simulink model "MIL4L3_SW6_V1_20220211"  (R2018b)
settings: Solver=FixedStepAuto  StartTime=0.0  StopTime=inf  FixedStep=0.001  RelTol=1e-3
PreLoadFcn:
  | A0_MILtest;
undefined symbols (not defined in the file or in its folder): Clb_ICADirect_LaneDisp_StateFive, Clb_ICADirect_LaneDisp_StateFour, Clb_ICADirect_LaneDisp_StateOne, Clb_ICADirect_LaneDisp_StateThree, Clb_ICADirect_LaneDisp_StateTwo, Clb_ICADirect_LaneDisp_StateZero, Clb_ICADirect_LaneDispSW, Clb_ICADirect_TrnLghtsCom_Switch, Clb_ICADirect_TrnLghtsCom_Value, Clb_ICADirect_TrnLghtsCrtl_Inhb, IMAP_Clb_ACU_Driver_Belt, IMAP_Clb_ACU_Driver_Belt_Over, IMAP_Clb_ACU_Passenger_Belt, IMAP_Clb_ACU_Passenger_Belt_Over, IMAP_Clb_ACU_RearLeft_Belt, IMAP_Clb_ACU_RearLeft_Belt_Over, IMAP_Clb_ACU_RearMiddle_Belt, IMAP_Clb_ACU_RearMiddle_Belt_Over, IMAP_Clb_ACU_RearRight_Belt, IMAP_Clb_ACU_RearRight_Belt_Over, IMAP_Clb_AEB_Switch, IMAP_Clb_AEB_Switch_Over, IMAP_Clb_ALC_TLC_Mode, IMAP_Clb_ALC_TLC_Mode_Over, IMAP_Clb_BCM_Battery_Voltage, IMAP_Clb_BCM_Battery_Voltage_Over, IMAP_Clb_BCM_BrakeLamp_State, IMAP_Clb_BCM_BrakeLamp_State_Over, IMAP_Clb_BCM_CHMSL_Status, IMAP_Clb_BCM_CHMSL_Status_Over, IMAP_Clb_BCM_Door_Lock_State, IMAP_Clb_BCM_Door_Lock_State_Over, IMAP_Clb_BCM_FrontWiper_State, IMAP_Clb_BCM_FrontWiper_State_Over, IMAP_Clb_BCM_FrontWiper_Switch, IMAP_Clb_BCM_FrontWiper_Switch_Over, IMAP_Clb_BCM_HazardLamp, IMAP_Clb_BCM_HazardLamp_Over, IMAP_Clb_BCM_HazardLamp_Switch, IMAP_Clb_BCM_HazardLamp_Switch_Over, IMAP_Clb_BCM_HighBeam_State, IMAP_Clb_BCM_HighBeam_State_Over, IMAP_Clb_BCM_Ignition_State, IMAP_Clb_BCM_Ignition_State_Over, IMAP_Clb_BCM_IHBC_Enabled, IMAP_Clb_BCM_IHBC_Enabled_Over, IMAP_Clb_BCM_Left_Light, IMAP_Clb_BCM_Left_Light_Over, IMAP_Clb_BCM_LeftTurn_Switch, IMAP_Clb_BCM_LeftTurn_Switch_Over, IMAP_Clb_BCM_LF_Door_State, IMAP_Clb_BCM_LF_Door_State_Over, IMAP_Clb_BCM_LowBeam_State, IMAP_Clb_BCM_LowBeam_State_Over, IMAP_Clb_BCM_LR_Door_State, IMAP_Clb_BCM_LR_Door_State_Over, IMAP_Clb_BCM_RF_Door_State, IMAP_Clb_BCM_RF_Door_State_Over, IMAP_Clb_BCM_Right_Light, IMAP_Clb_BCM_Right_Light_Over ... (+547)
libraries: CarMaker4SL x2153, simulink x292, dspstat3 x3, canmsglib x2, simulink_extras x1
(part 14 of 52)

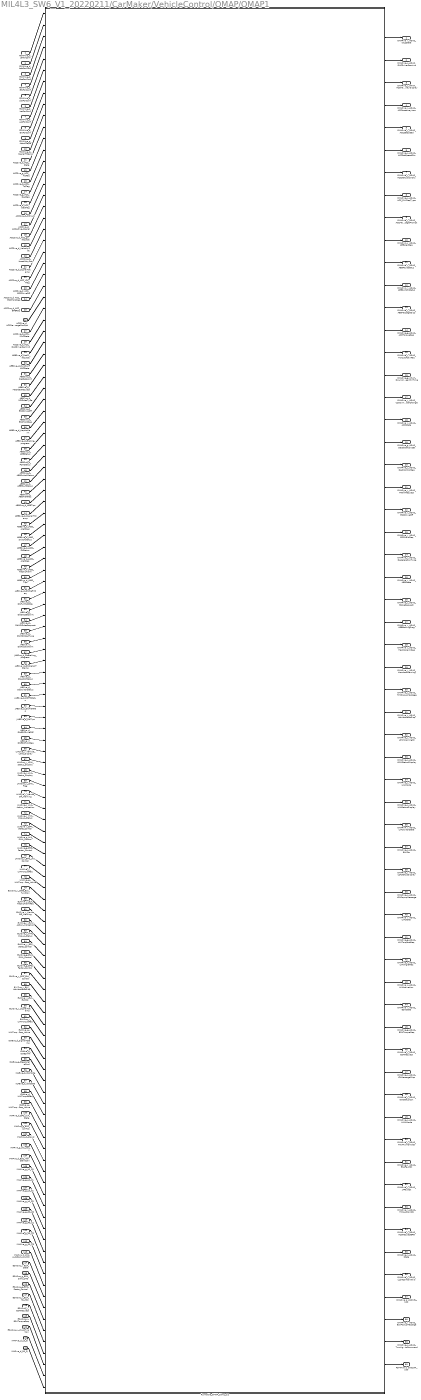
== system MIL4L3_SW6_V1_20220211/CarMaker/VehicleControl/OMAP/OMAP1 ==
  FDMMve_d_JaFcnConf : Inport  OutDataTypeStr=UInt16  PortDimensions=1
  FDMMve_d_AebFcnConf : Inport  Port=2  OutDataTypeStr=UInt16  PortDimensions=1
  FDMMve_d_EsaFcnConf : Inport  Port=3  OutDataTypeStr=UInt16  PortDimensions=1
  FDMMve_d_ElkFcnConf : Inport  Port=4  OutDataTypeStr=UInt16  PortDimensions=1
  FDMMve_d_LkaFcnConf : Inport  Port=5  OutDataTypeStr=UInt16  PortDimensions=1
  FDMMve_d_IcaFcnConf : Inport  Port=6  OutDataTypeStr=UInt16  PortDimensions=1
  FDMMve_d_AccFcnConf : Inport  Port=7  OutDataTypeStr=UInt16  PortDimensions=1
  FDMMve_d_EwFcnConf : Inport  Port=8  OutDataTypeStr=UInt16  PortDimensions=1
  FDMMve_g_Adas2Fapa : Inport  Port=9  OutDataTypeStr=UInt32  PortDimensions=1
  FDMMve_d_SignalTStamp : Inport  Port=10  OutDataTypeStr=UInt16  PortDimensions=1
  ACCSve_d_ACC_State : Inport  Port=11  OutDataTypeStr=UInt16  PortDimensions=1
  ACCSve_g_ACC_TqReq : Inport  Port=12  OutDataTypeStr=T_M_Nm_Float32  PortDimensions=1
  ACCSve_d_ACC_TqFlag : Inport  Port=13  OutDataTypeStr=UInt16  PortDimensions=1
  ACCSve_g_ACC_DecReq : Inport  Port=14  OutDataTypeStr=T_M_Nm_Float32  PortDimensions=1
  ACCSve_d_ACC_DecFlag : Inport  Port=15  OutDataTypeStr=UInt16  PortDimensions=1
  ACCSve_d_CIPV_ID : Inport  Port=16  OutDataTypeStr=UInt16  PortDimensions=1
  ACCSve_d_ACCActive_Signal : Inport  Port=17  OutDataTypeStr=UInt16  PortDimensions=1
  ACCSve_d_ACC_go_request : Inport  Port=18  OutDataTypeStr=UInt16  PortDimensions=1
  ACCSve_d_VelocitySet : Inport  Port=19  OutDataTypeStr=UInt16  PortDimensions=1
  ACCSve_d_HeadWaySet : Inport  Port=20  OutDataTypeStr=UInt16  PortDimensions=1
  ACCSve_d_SignalTStamp : Inport  Port=21  OutDataTypeStr=UInt16  PortDimensions=1
  ACCSve_d_ACC_ICA_Flag : Inport  Port=22  OutDataTypeStr=UInt16  PortDimensions=1
  ACCSve_d_ACC_ESCDriveOff : Inport  Port=23  OutDataTypeStr=UInt16  PortDimensions=1
  ACCSve_d_ACC_ESCHoldReq : Inport  Port=24  OutDataTypeStr=UInt16  PortDimensions=1
  ACCSve_d_ACC_EPBReq : Inport  Port=25  OutDataTypeStr=UInt16  PortDimensions=1
  ACCSve_d_ACCMessagePrompt : Inport  Port=26  OutDataTypeStr=UInt16
  ACCSve_d_ACC_ISLCState : Inport  Port=27  OutDataTypeStr=UInt16  PortDimensions=1
  ACCSve_d_ACC_ISLCDriverRemind : Inport  Port=28  OutDataTypeStr=UInt16  PortDimensions=1
  AEBSve_d_Prefill_request : Inport  Port=29  OutDataTypeStr=UInt16  PortDimensions=1
  AEBSve_d_functionFARCState : Inport  Port=30  OutDataTypeStr=UInt16  PortDimensions=1
  AEBSve_g_DecSetpoint : Inport  Port=31  OutDataTypeStr=T_M_Nm_Float32  PortDimensions=1
  AEBSve_d_MDDdecRequest : Inport  Port=32  OutDataTypeStr=UInt16  PortDimensions=1
  AEBSve_d_MDDdecType : Inport  Port=33  OutDataTypeStr=UInt16  PortDimensions=1
  AEBSve_d_ESCDriveOff : Inport  Port=34  OutDataTypeStr=UInt16  PortDimensions=1
  AEBSve_d_ESCHoldReq : Inport  Port=35  OutDataTypeStr=UInt16  PortDimensions=1
  AEBSve_d_HapticAlarm : Inport  Port=36  OutDataTypeStr=UInt16  PortDimensions=1
  AEBSve_d_Braking_progress : Inport  Port=37  OutDataTypeStr=UInt16  PortDimensions=1
  AEBSve_d_AEBStatus : Inport  Port=38  OutDataTypeStr=UInt16  PortDimensions=1
  AEBSve_d_FCWStatus : Inport  Port=39  OutDataTypeStr=UInt16  PortDimensions=1
  AEBSve_d_AEBSwitchStatus : Inport  Port=40  OutDataTypeStr=UInt16  PortDimensions=1
  AEBSve_d_AEBFaultStatus : Inport  Port=41  OutDataTypeStr=UInt16  PortDimensions=1
  AEBSve_d_AEBAlertReq : Inport  Port=42  OutDataTypeStr=UInt16  PortDimensions=1
  AEBSve_d_AEBTips : Inport  Port=43  OutDataTypeStr=UInt16  PortDimensions=1
  AEBSve_d_SignalTStamp : Inport  Port=44  OutDataTypeStr=UInt16  PortDimensions=1
  AEBSve_d_JABS_AlertSign : Inport  Port=45  OutDataTypeStr=UInt16  PortDimensions=1
  AEBSve_d_JABS_SwitchStatus : Inport  Port=46  OutDataTypeStr=UInt16  PortDimensions=1
  AEBSve_d_JABS_FltStatus : Inport  Port=47  OutDataTypeStr=UInt16  PortDimensions=1
  AEBSve_d_JABS_AlertReq : Inport  Port=48  OutDataTypeStr=UInt16  PortDimensions=1
  AEBSve_d_JABS_HapticAlarm : Inport  Port=49  OutDataTypeStr=UInt16  PortDimensions=1
  AEBSve_d_JABS_Tips : Inport  Port=50  OutDataTypeStr=UInt16  PortDimensions=1
  JABSve_d_DbPrefillReq : Inport  Port=51  OutDataTypeStr=UInt16  PortDimensions=1
  JABSve_d_DbFunFARCSta : Inport  Port=52  OutDataTypeStr=UInt16  PortDimensions=1
  JABSve_g_DbDecSetpoint : Inport  Port=53  OutDataTypeStr=T_M_Nm_Float32  PortDimensions=1
  JABSve_d_DbMDDdecRequest : Inport  Port=54  OutDataTypeStr=UInt16  PortDimensions=1
  JABSve_d_DbMDDdecType : Inport  Port=55  OutDataTypeStr=UInt16  PortDimensions=1
  JABSve_d_DbHapticAlarm : Inport  Port=56  OutDataTypeStr=UInt16  PortDimensions=1
  JABSve_d_DbBraking_progress : Inport  Port=57  OutDataTypeStr=UInt16  PortDimensions=1
  JABSve_d_DbSignalTStamp : Inport  Port=58  OutDataTypeStr=UInt16  PortDimensions=1
  JABSve_d_DbJACWStatus : Inport  Port=59  OutDataTypeStr=UInt16  PortDimensions=1
  JABSve_d_DbSwitchStatus : Inport  Port=60  OutDataTypeStr=UInt16  PortDimensions=1
  JABSve_d_DbFltStatus : Inport  Port=61  OutDataTypeStr=UInt16  PortDimensions=1
  JABSve_d_DbAlertReq : Inport  Port=62  OutDataTypeStr=UInt16  PortDimensions=1
  JABSve_d_DbTips : Inport  Port=63  OutDataTypeStr=UInt16  PortDimensions=1
  JABSve_d_DbESCDriveOff : Inport  Port=64  OutDataTypeStr=UInt16  PortDimensions=1
  JABSve_d_DbESCHoldReq : Inport  Port=65  OutDataTypeStr=UInt16  PortDimensions=1
  LKASve_y_Vehicle_Lane_Display : Inport  Port=66  OutDataTypeStr=UInt8  PortDimensions=1
  LKASve_y_LDW_Status_Display : Inport  Port=67  OutDataTypeStr=UInt8  PortDimensions=1
  LKASve_y_LKA_Status_Display : Inport  Port=68  OutDataTypeStr=UInt8  PortDimensions=1
  LKASve_y_LDW_Flag : Inport  Port=69  OutDataTypeStr=UInt8  PortDimensions=1
  LKASve_y_Hands_Off_Warning : Inport  Port=70  OutDataTypeStr=UInt8  PortDimensions=1
  LKASve_y_LKA_Action_Indication : Inport  Port=71  OutDataTypeStr=UInt8  PortDimensions=1
  LKASve_y_HMI_Popup_Status : Inport  Port=72  OutDataTypeStr=UInt8  PortDimensions=1
  LKASve_y_EPS_State_Control : Inport  Port=73  OutDataTypeStr=UInt8  PortDimensions=1
  LKASve_g_LKA_SWA_Control : Inport  Port=74  OutDataTypeStr=T_M_Nm_Float32  PortDimensions=1
  LKASve_g_EPS_Factor_Control : Inport  Port=75  OutDataTypeStr=T_M_Nm_Float32  PortDimensions=1
  LKASve_y_EPS_LKA_Control : Inport  Port=76  OutDataTypeStr=UInt8  PortDimensions=1
  LKASve_y_LKATorqueReq : Inport  Port=77  OutDataTypeStr=UInt8  PortDimensions=1
  LKASve_g_LKATorqueReq_Value : Inport  Port=78  OutDataTypeStr=T_M_Nm_Float32  PortDimensions=1
  ELKSve_y_state_ELK_function : Inport  Port=79  OutDataTypeStr=UInt8  PortDimensions=1
  ELKSve_y_ELK_HapticAlarmReq : Inport  Port=80  OutDataTypeStr=UInt8  PortDimensions=1
  ELKSve_y_Hands_Off_Warning : Inport  Port=81  OutDataTypeStr=UInt8  PortDimensions=1
  ELKSve_y_ELK_Action_Indication : Inport  Port=82  OutDataTypeStr=UInt8  PortDimensions=1
  ELKSve_y_HMI_Popup_Status : Inport  Port=83  OutDataTypeStr=UInt8  PortDimensions=1
  ELKSve_y_EPS_State_Control : Inport  Port=84  OutDataTypeStr=UInt8  PortDimensions=1
  ELKSve_g_ELK_SWA_Control : Inport  Port=85  OutDataTypeStr=T_M_Nm_Float32  PortDimensions=1
  ELKSve_g_EPS_Factor_Control : Inport  Port=86  OutDataTypeStr=T_M_Nm_Float32  PortDimensions=1
  ELKSve_y_EPS_ELK_Control : Inport  Port=87  OutDataTypeStr=UInt8  PortDimensions=1
  ELKSve_y_ELK_VehicleLaneDisp : Inport  Port=88  OutDataTypeStr=UInt8  PortDimensions=1
  ELKSve_y_ELK_ELKSts : Inport  Port=89  OutDataTypeStr=UInt8  PortDimensions=1
  ELKSve_y_SignalTStamp : Inport  Port=90  OutDataTypeStr=UInt8  PortDimensions=1
  ELKSve_y_LKATorqueReq : Inport  Port=91  OutDataTypeStr=UInt8  PortDimensions=1
  ELKSve_g_LKATorqueReq_Value : Inport  Port=92  OutDataTypeStr=T_M_Nm_Float32  PortDimensions=1
  ICABve_d_SignalTStamp : Inport  Port=93  OutDataTypeStr=UInt16  PortDimensions=1
  ICABva_d_ICAB2HMI : Inport  Port=94  OutDataTypeStr=UInt16  PortDimensions=20
  ICABve_g_SteerAngleCmd : Inport  Port=95  OutDataTypeStr=T_M_Nm_Float32  PortDimensions=1
  ICABve_d_ICAMode : Inport  Port=96  OutDataTypeStr=UInt16  PortDimensions=1
  ICABve_d_ICAState : Inport  Port=97  OutDataTypeStr=UInt16  PortDimensions=1
  ICABve_d_LKATorqueReq : Inport  Port=98  OutDataTypeStr=UInt16  PortDimensions=1
  ICABve_g_LKATorqueReq_Value : Inport  Port=99  OutDataTypeStr=T_M_Nm_Float32  PortDimensions=1
  IMAPve_d_EPS_LKA_State : Inport  Port=100  OutDataTypeStr=UInt16  PortDimensions=1
  IMAPve_g_ESC_LonAcc : Inport  Port=101  OutDataTypeStr=T_M_Nm_Float32  PortDimensions=1
  IMAPva_d_obj_id : Inport  Port=102  OutDataTypeStr=UInt16  PortDimensions=40
  IMAPva_g_obj_pos_x : Inport  Port=103  OutDataTypeStr=T_M_Nm_Float32  PortDimensions=40
  IMAPve_d_ESC_Veh_Standstill : Inport  Port=104  OutDataTypeStr=UInt16  PortDimensions=1
  IMAPve_g_L0_C0 : Inport  Port=105  OutDataTypeStr=T_M_Nm_Float32  PortDimensions=1
  IMAPve_g_L0_C1 : Inport  Port=106  OutDataTypeStr=T_M_Nm_Float32  PortDimensions=1
  IMAPve_g_L0_C2 : Inport  Port=107  OutDataTypeStr=T_M_Nm_Float32  PortDimensions=1
  IMAPve_g_L0_C3 : Inport  Port=108  OutDataTypeStr=T_M_Nm_Float32  PortDimensions=1
  IMAPve_g_R0_C0 : Inport  Port=109  OutDataTypeStr=T_M_Nm_Float32  PortDimensions=1
  IMAPve_g_R0_C1 : Inport  Port=110  OutDataTypeStr=T_M_Nm_Float32  PortDimensions=1
  IMAPve_g_R0_C2 : Inport  Port=111  OutDataTypeStr=T_M_Nm_Float32  PortDimensions=1
  IMAPve_g_R0_C3 : Inport  Port=112  OutDataTypeStr=T_M_Nm_Float32  PortDimensions=1
  IMAPve_d_APA_AutoPark_WorkSt : Inport  Port=113  OutDataTypeStr=UInt16  PortDimensions=1
  ESASve_y_ESA_State : Inport  Port=114  OutDataTypeStr=UInt8
  ESASve_g_ESA_SWA_CMD : Inport  Port=115  OutDataTypeStr=T_M_Nm_Float32
  ESASve_g_EPS_Factor_Control : Inport  Port=116  OutDataTypeStr=T_M_Nm_Float32
  ESASve_y_ESA_FaultSt : Inport  Port=117  OutDataTypeStr=UInt8
  ESASve_y_ESARequest : Inport  Port=118  OutDataTypeStr=UInt8
  ESASve_y_ESATorqueReq : Inport  Port=119  OutDataTypeStr=T_M_Nm_Float32
  ESASve_y_LKAActivation : Inport  Port=120  OutDataTypeStr=UInt8
  IMAPve_d_L0_Q : Inport  Port=121  OutDataTypeStr=UInt16
  IMAPve_d_R0_Q : Inport  Port=122  OutDataTypeStr=UInt16
  Runnable_OMAP_10ms_sys : Subsystem
  OMAPve_y_ADAS_ISLCState : Outport  OutDataTypeStr=UInt8  PortDimensions=1
  OMAPve_y_ADAS_ISLCDriverRemind : Outport  Port=2  OutDataTypeStr=UInt8  PortDimensions=1
  OMAPve_y_ADAS_ACCHeadwayDisplay : Outport  Port=3  OutDataTypeStr=UInt8  PortDimensions=1
  OMAPve_y_ADAS_ACCHeadwayIcon : Outport  Port=4  OutDataTypeStr=UInt8  PortDimensions=1
  OMAPve_y_ADAS_ACCSetSpeed : Outport  Port=5  OutDataTypeStr=UInt8  PortDimensions=1
  OMAPve_y_ADAS_ACCSetSpeedDis : Outport  Port=6  OutDataTypeStr=UInt8  PortDimensions=1
  OMAPve_y_ADAS_ACCStatusIconDis : Outport  Port=7  OutDataTypeStr=UInt8  PortDimensions=1
  OMAPve_y_ADAS_ACC_RVVReqType : Outport  Port=8  OutDataTypeStr=UInt8  PortDimensions=1
  OMAPve_y_ADAS_ACCMessagePrompt : Outport  Port=9  OutDataTypeStr=UInt8  PortDimensions=1
  OMAPve_y_ADAS_AEBAlertReq : Outport  Port=10  OutDataTypeStr=UInt8  PortDimensions=1
  OMAPve_y_ADAS_AEBFaultStatus : Outport  Port=11  OutDataTypeStr=UInt8  PortDimensions=1
  OMAPve_y_ADAS_AEBSwitchStatus : Outport  Port=12  OutDataTypeStr=UInt8  PortDimensions=1
  OMAPve_y_ADAS_AEBMassageDisp : Outport  Port=13  OutDataTypeStr=UInt8  PortDimensions=1
  OMAPve_g_ADAS_ACCTorqueReq : Outport  Port=14  OutDataTypeStr=T_M_Nm_Float32  PortDimensions=1
  OMAPve_y_ADAS_TorqueActivReq : Outport  Port=15  OutDataTypeStr=UInt8  PortDimensions=1
  OMAPve_g_ADAS_DownorUpGearMinTime : Outport  Port=16  OutDataTypeStr=T_M_Nm_Float32  PortDimensions=1
  OMAPve_y_ADAS_UpDownGearChange : Outport  Port=17  OutDataTypeStr=UInt8  PortDimensions=1
  OMAPve_y_ADAS_ACCState : Outport  Port=18  OutDataTypeStr=UInt8  PortDimensions=1
  OMAPve_g_ADAS_DecelerationSet : Outport  Port=19  OutDataTypeStr=T_M_Nm_Float32  PortDimensions=1
  OMAPve_y_ADAS_DeclControlReq : Outport  Port=20  OutDataTypeStr=UInt8  PortDimensions=1
  OMAPve_y_ADAS_PrefillRequest : Outport  Port=21  OutDataTypeStr=UInt8  PortDimensions=1
  OMAPve_y_ADAS_ESCDriveOff : Outport  Port=22  OutDataTypeStr=UInt8  PortDimensions=1
  OMAPve_y_ADAS_ESCHoldReq : Outport  Port=23  OutDataTypeStr=UInt8  PortDimensions=1
  OMAPve_y_ADAS_DecelerationType : Outport  Port=24  OutDataTypeStr=UInt8  PortDimensions=1
  OMAPve_y_ADAS_AEBState : Outport  Port=25  OutDataTypeStr=UInt8  PortDimensions=1
  OMAPve_y_ADAS_BrakeRequest : Outport  Port=26  OutDataTypeStr=UInt8  PortDimensions=1
  OMAPve_y_ADAS_AEBBrakingProg : Outport  Port=27  OutDataTypeStr=UInt8  PortDimensions=1
  OMAPve_y_ADAS_HapticAlarmReq : Outport  Port=28  OutDataTypeStr=UInt8  PortDimensions=1
  OMAPve_y_ADAS_Handsoffwarning : Outport  Port=29  OutDataTypeStr=UInt8  PortDimensions=1
  OMAPve_y_ADAS_HMIPopupMassage : Outport  Port=30  OutDataTypeStr=UInt8  PortDimensions=1
  OMAPve_y_ADAS_VehicleLaneDisp : Outport  Port=31  OutDataTypeStr=UInt8  PortDimensions=1
  OMAPve_y_ADAS_LDWWarningSt : Outport  Port=32  OutDataTypeStr=UInt8  PortDimensions=1
  OMAPve_y_ADAS_LDWStatusDisplay : Outport  Port=33  OutDataTypeStr=UInt8  PortDimensions=1
  OMAPve_y_ADAS_LKAMode : Outport  Port=34  OutDataTypeStr=UInt8  PortDimensions=1
  OMAPve_y_ADAS_LKAStatusDisplay : Outport  Port=35  OutDataTypeStr=UInt8  PortDimensions=1
  OMAPve_y_ADAS_LKASwitchState : Outport  Port=36  OutDataTypeStr=UInt8  PortDimensions=1
  OMAPve_y_ADAS_ELKSts : Outport  Port=37  OutDataTypeStr=UInt8  PortDimensions=1
  OMAPve_y_ADAS_LCAStatusDisplay : Outport  Port=38  OutDataTypeStr=UInt8  PortDimensions=1
  OMAPve_y_ADAS_LCAPopupMessage : Outport  Port=39  OutDataTypeStr=UInt8  PortDimensions=1
  OMAPve_y_ADAS_LKAState : Outport  Port=40  OutDataTypeStr=UInt8  PortDimensions=1
  OMAPve_g_ADAS_LKATorqFactReq : Outport  Port=41  OutDataTypeStr=T_M_Nm_Float32  PortDimensions=1
  OMAPve_g_ADAS_LKAAngleReq : Outport  Port=42  OutDataTypeStr=T_M_Nm_Float32  PortDimensions=1
  OMAPve_y_ADAS_LKAActivation : Outport  Port=43  OutDataTypeStr=UInt8  PortDimensions=1
  OMAPve_y_ADAS_ESAState : Outport  Port=44  OutDataTypeStr=UInt8  PortDimensions=1
  OMAPve_g_ADAS_ESATorqueReq : Outport  Port=45  OutDataTypeStr=T_M_Nm_Float32  PortDimensions=1
  OMAPve_y_ADAS_ESARequest : Outport  Port=46  OutDataTypeStr=UInt8  PortDimensions=1
  OMAPve_y_ADAS_ICAMassageDisp : Outport  Port=47  OutDataTypeStr=UInt8  PortDimensions=1
  OMAPve_y_ADAS_ICAStatusIcon : Outport  Port=48  OutDataTypeStr=UInt8  PortDimensions=1
  OMAPve_y_ADAS_HWAMode : Outport  Port=49  OutDataTypeStr=UInt8  PortDimensions=1
  OMAPve_y_ADAS_HWATurnOnIdctr : Outport  Port=50  OutDataTypeStr=UInt8  PortDimensions=1
  OMAPve_y_ADAS_ESAFaultSt : Outport  Port=51  OutDataTypeStr=UInt8  PortDimensions=1
  OMAPve_y_ADAS_JAFaultSt : Outport  Port=52  OutDataTypeStr=UInt8  PortDimensions=1
  OMAPve_y_ADAS_HWAActionSts : Outport  Port=53  OutDataTypeStr=UInt8  PortDimensions=1
  OMAPve_y_ADAS_ACCRequestEPB : Outport  Port=54  OutDataTypeStr=UInt8  PortDimensions=1
  OMAPve_y_ADAS_State : Outport  Port=55  OutDataTypeStr=UInt8  PortDimensions=1
  OMAPve_y_ADAS_LightControlValid : Outport  Port=56  OutDataTypeStr=UInt8  PortDimensions=1
  OMAPve_g_ob019L_100 : Outport  Port=57  OutDataTypeStr=UInt32  PortDimensions=1
  OMAPve_y_ADAS_ELKPopupMessage : Outport  Port=58  OutDataTypeStr=UInt8
  OMAPve_y_ADAS_TurnLightsCommand : Outport  Port=59  OutDataTypeStr=UInt8
  FDMMve_g_ob019H_100 : Outport  Port=60  OutDataTypeStr=UInt32
  wires:
  JABSve_d_DbTips/1 -> Runnable_OMAP_10ms_sys/63(JABSve_d_DbTips)
  ELKSve_y_ELK_VehicleLaneDisp/1 -> Runnable_OMAP_10ms_sys/88(ELKSve_y_ELK_VehicleLaneDisp)
  Runnable_OMAP_10ms_sys/39(OMAPve_y_ADAS_LCAPopupMessage) -> OMAPve_y_ADAS_LCAPopupMessage/1
  LKASve_g_LKATorqueReq_Value/1 -> Runnable_OMAP_10ms_sys/78(LKASve_g_LKATorqueReq_Value)
  ACCSve_d_SignalTStamp/1 -> Runnable_OMAP_10ms_sys/21(ACCSve_d_SignalTStamp)
  Runnable_OMAP_10ms_sys/18(OMAPve_y_ADAS_ACCState) -> OMAPve_y_ADAS_ACCState/1
  Runnable_OMAP_10ms_sys/24(OMAPve_y_ADAS_DecelerationType) -> OMAPve_y_ADAS_DecelerationType/1
  ACCSve_d_ACC_ISLCDriverRemind/1 -> Runnable_OMAP_10ms_sys/28(ACCSve_d_ACC_ISLCDriverRemind)
  AEBSve_d_MDDdecType/1 -> Runnable_OMAP_10ms_sys/33(AEBSve_d_MDDdecType)
  LKASve_y_LKA_Status_Display/1 -> Runnable_OMAP_10ms_sys/68(LKASve_y_LKA_Status_Display)
  Runnable_OMAP_10ms_sys/17(OMAPve_y_ADAS_UpDownGearChange) -> OMAPve_y_ADAS_UpDownGearChange/1
  Runnable_OMAP_10ms_sys/60(FDMMve_g_ob019H_100) -> FDMMve_g_ob019H_100/1
  Runnable_OMAP_10ms_sys/6(OMAPve_y_ADAS_ACCSetSpeedDis) -> OMAPve_y_ADAS_ACCSetSpeedDis/1
  IMAPve_d_L0_Q/1 -> Runnable_OMAP_10ms_sys/121(IMAPve_d_L0_Q)
  Runnable_OMAP_10ms_sys/58(OMAPve_y_ADAS_ELKPopupMessage) -> OMAPve_y_ADAS_ELKPopupMessage/1
  Runnable_OMAP_10ms_sys/11(OMAPve_y_ADAS_AEBFaultStatus) -> OMAPve_y_ADAS_AEBFaultStatus/1
  ESASve_g_ESA_SWA_CMD/1 -> Runnable_OMAP_10ms_sys/115(ESASve_g_ESA_SWA_CMD)
  Runnable_OMAP_10ms_sys/41(OMAPve_g_ADAS_LKATorqFactReq) -> OMAPve_g_ADAS_LKATorqFactReq/1
  Runnable_OMAP_10ms_sys/45(OMAPve_g_ADAS_ESATorqueReq) -> OMAPve_g_ADAS_ESATorqueReq/1
  ICABve_g_LKATorqueReq_Value/1 -> Runnable_OMAP_10ms_sys/99(ICABve_g_LKATorqueReq_Value)
  Runnable_OMAP_10ms_sys/46(OMAPve_y_ADAS_ESARequest) -> OMAPve_y_ADAS_ESARequest/1
  ESASve_y_ESARequest/1 -> Runnable_OMAP_10ms_sys/118(ESASve_y_ESARequest)
  ELKSve_y_Hands_Off_Warning/1 -> Runnable_OMAP_10ms_sys/81(ELKSve_y_Hands_Off_Warning)
  Runnable_OMAP_10ms_sys/20(OMAPve_y_ADAS_DeclControlReq) -> OMAPve_y_ADAS_DeclControlReq/1
  IMAPve_g_L0_C3/1 -> Runnable_OMAP_10ms_sys/108(IMAPve_g_L0_C3)
  ESASve_y_LKAActivation/1 -> Runnable_OMAP_10ms_sys/120(ESASve_y_LKAActivation)
  JABSve_d_DbHapticAlarm/1 -> Runnable_OMAP_10ms_sys/56(JABSve_d_DbHapticAlarm)
  ESASve_y_ESA_State/1 -> Runnable_OMAP_10ms_sys/114(ESASve_y_ESA_State)
  ESASve_y_ESA_FaultSt/1 -> Runnable_OMAP_10ms_sys/117(ESASve_y_ESA_FaultSt)
  ESASve_y_ESATorqueReq/1 -> Runnable_OMAP_10ms_sys/119(ESASve_y_ESATorqueReq)
  IMAPve_d_ESC_Veh_Standstill/1 -> Runnable_OMAP_10ms_sys/104(IMAPve_d_ESC_Veh_Standstill)
  Runnable_OMAP_10ms_sys/52(OMAPve_y_ADAS_JAFaultSt) -> OMAPve_y_ADAS_JAFaultSt/1
  Runnable_OMAP_10ms_sys/34(OMAPve_y_ADAS_LKAMode) -> OMAPve_y_ADAS_LKAMode/1
  ACCSve_d_ACC_go_request/1 -> Runnable_OMAP_10ms_sys/18(ACCSve_d_ACC_go_request)
  Runnable_OMAP_10ms_sys/50(OMAPve_y_ADAS_HWATurnOnIdctr) -> OMAPve_y_ADAS_HWATurnOnIdctr/1
  ELKSve_g_LKATorqueReq_Value/1 -> Runnable_OMAP_10ms_sys/92(ELKSve_g_LKATorqueReq_Value)
  Runnable_OMAP_10ms_sys/21(OMAPve_y_ADAS_PrefillRequest) -> OMAPve_y_ADAS_PrefillRequest/1
  Runnable_OMAP_10ms_sys/57(OMAPve_g_ob019L_100) -> OMAPve_g_ob019L_100/1
  Runnable_OMAP_10ms_sys/55(OMAPve_y_ADAS_State) -> OMAPve_y_ADAS_State/1
  LKASve_y_LKATorqueReq/1 -> Runnable_OMAP_10ms_sys/77(LKASve_y_LKATorqueReq)
  ACCSve_d_ACC_ISLCState/1 -> Runnable_OMAP_10ms_sys/27(ACCSve_d_ACC_ISLCState)
  Runnable_OMAP_10ms_sys/26(OMAPve_y_ADAS_BrakeRequest) -> OMAPve_y_ADAS_BrakeRequest/1
  Runnable_OMAP_10ms_sys/37(OMAPve_y_ADAS_ELKSts) -> OMAPve_y_ADAS_ELKSts/1
  ELKSve_y_ELK_Action_Indication/1 -> Runnable_OMAP_10ms_sys/82(ELKSve_y_ELK_Action_Indication)
  ELKSve_g_EPS_Factor_Control/1 -> Runnable_OMAP_10ms_sys/86(ELKSve_g_EPS_Factor_Control)
  JABSve_d_DbFltStatus/1 -> Runnable_OMAP_10ms_sys/61(JABSve_d_DbFltStatus)
  ICABve_d_ICAMode/1 -> Runnable_OMAP_10ms_sys/96(ICABve_d_ICAMode)
  ICABve_g_SteerAngleCmd/1 -> Runnable_OMAP_10ms_sys/95(ICABve_g_SteerAngleCmd)
  AEBSve_d_JABS_AlertReq/1 -> Runnable_OMAP_10ms_sys/48(AEBSve_d_JABS_AlertReq)
  LKASve_y_EPS_State_Control/1 -> Runnable_OMAP_10ms_sys/73(LKASve_y_EPS_State_Control)
  Runnable_OMAP_10ms_sys/5(OMAPve_y_ADAS_ACCSetSpeed) -> OMAPve_y_ADAS_ACCSetSpeed/1
  IMAPva_d_obj_id/1 -> Runnable_OMAP_10ms_sys/102(IMAPva_d_obj_id)
  Runnable_OMAP_10ms_sys/23(OMAPve_y_ADAS_ESCHoldReq) -> OMAPve_y_ADAS_ESCHoldReq/1
  Runnable_OMAP_10ms_sys/12(OMAPve_y_ADAS_AEBSwitchStatus) -> OMAPve_y_ADAS_AEBSwitchStatus/1
  FDMMve_d_EsaFcnConf/1 -> Runnable_OMAP_10ms_sys/3(FDMMve_d_EsaFcnConf)
  Runnable_OMAP_10ms_sys/4(OMAPve_y_ADAS_ACCHeadwayIcon) -> OMAPve_y_ADAS_ACCHeadwayIcon/1
  ESASve_g_EPS_Factor_Control/1 -> Runnable_OMAP_10ms_sys/116(ESASve_g_EPS_Factor_Control)
  AEBSve_d_JABS_FltStatus/1 -> Runnable_OMAP_10ms_sys/47(AEBSve_d_JABS_FltStatus)
  IMAPve_d_R0_Q/1 -> Runnable_OMAP_10ms_sys/122(IMAPve_d_R0_Q)
  Runnable_OMAP_10ms_sys/40(OMAPve_y_ADAS_LKAState) -> OMAPve_y_ADAS_LKAState/1
  ACCSve_g_ACC_TqReq/1 -> Runnable_OMAP_10ms_sys/12(ACCSve_g_ACC_TqReq)
  ELKSve_y_ELK_HapticAlarmReq/1 -> Runnable_OMAP_10ms_sys/80(ELKSve_y_ELK_HapticAlarmReq)
  IMAPve_g_R0_C0/1 -> Runnable_OMAP_10ms_sys/109(IMAPve_g_R0_C0)
  ELKSve_y_LKATorqueReq/1 -> Runnable_OMAP_10ms_sys/91(ELKSve_y_LKATorqueReq)
  Runnable_OMAP_10ms_sys/28(OMAPve_y_ADAS_HapticAlarmReq) -> OMAPve_y_ADAS_HapticAlarmReq/1
  FDMMve_d_LkaFcnConf/1 -> Runnable_OMAP_10ms_sys/5(FDMMve_d_LkaFcnConf)
  AEBSve_d_AEBTips/1 -> Runnable_OMAP_10ms_sys/43(AEBSve_d_AEBTips)
  Runnable_OMAP_10ms_sys/10(OMAPve_y_ADAS_AEBAlertReq) -> OMAPve_y_ADAS_AEBAlertReq/1
  AEBSve_d_ESCHoldReq/1 -> Runnable_OMAP_10ms_sys/35(AEBSve_d_ESCHoldReq)
  Runnable_OMAP_10ms_sys/59(OMAPve_y_ADAS_TurnLightsCommand) -> OMAPve_y_ADAS_TurnLightsCommand/1
  Runnable_OMAP_10ms_sys/8(OMAPve_y_ADAS_ACC_RVVReqType) -> OMAPve_y_ADAS_ACC_RVVReqType/1
  IMAPve_d_APA_AutoPark_WorkSt/1 -> Runnable_OMAP_10ms_sys/113(IMAPve_d_APA_AutoPark_WorkSt)
  FDMMve_d_AebFcnConf/1 -> Runnable_OMAP_10ms_sys/2(FDMMve_d_AebFcnConf)
  ICABva_d_ICAB2HMI/1 -> Runnable_OMAP_10ms_sys/94(ICABva_d_ICAB2HMI)
  Runnable_OMAP_10ms_sys/29(OMAPve_y_ADAS_Handsoffwarning) -> OMAPve_y_ADAS_Handsoffwarning/1
  Runnable_OMAP_10ms_sys/7(OMAPve_y_ADAS_ACCStatusIconDis) -> OMAPve_y_ADAS_ACCStatusIconDis/1
  FDMMve_d_IcaFcnConf/1 -> Runnable_OMAP_10ms_sys/6(FDMMve_d_IcaFcnConf)
  Runnable_OMAP_10ms_sys/14(OMAPve_g_ADAS_ACCTorqueReq) -> OMAPve_g_ADAS_ACCTorqueReq/1
  Runnable_OMAP_10ms_sys/44(OMAPve_y_ADAS_ESAState) -> OMAPve_y_ADAS_ESAState/1
  Runnable_OMAP_10ms_sys/30(OMAPve_y_ADAS_HMIPopupMassage) -> OMAPve_y_ADAS_HMIPopupMassage/1
  Runnable_OMAP_10ms_sys/54(OMAPve_y_ADAS_ACCRequestEPB) -> OMAPve_y_ADAS_ACCRequestEPB/1
  ACCSve_d_ACC_State/1 -> Runnable_OMAP_10ms_sys/11(ACCSve_d_ACC_State)
  AEBSve_d_JABS_SwitchStatus/1 -> Runnable_OMAP_10ms_sys/46(AEBSve_d_JABS_SwitchStatus)
  Runnable_OMAP_10ms_sys/13(OMAPve_y_ADAS_AEBMassageDisp) -> OMAPve_y_ADAS_AEBMassageDisp/1
  Runnable_OMAP_10ms_sys/49(OMAPve_y_ADAS_HWAMode) -> OMAPve_y_ADAS_HWAMode/1
  Runnable_OMAP_10ms_sys/47(OMAPve_y_ADAS_ICAMassageDisp) -> OMAPve_y_ADAS_ICAMassageDisp/1
  Runnable_OMAP_10ms_sys/43(OMAPve_y_ADAS_LKAActivation) -> OMAPve_y_ADAS_LKAActivation/1
  Runnable_OMAP_10ms_sys/27(OMAPve_y_ADAS_AEBBrakingProg) -> OMAPve_y_ADAS_AEBBrakingProg/1
  Runnable_OMAP_10ms_sys/42(OMAPve_g_ADAS_LKAAngleReq) -> OMAPve_g_ADAS_LKAAngleReq/1
  Runnable_OMAP_10ms_sys/16(OMAPve_g_ADAS_DownorUpGearMinTime) -> OMAPve_g_ADAS_DownorUpGearMinTime/1
  Runnable_OMAP_10ms_sys/31(OMAPve_y_ADAS_VehicleLaneDisp) -> OMAPve_y_ADAS_VehicleLaneDisp/1
  Runnable_OMAP_10ms_sys/25(OMAPve_y_ADAS_AEBState) -> OMAPve_y_ADAS_AEBState/1
  AEBSve_d_FCWStatus/1 -> Runnable_OMAP_10ms_sys/39(AEBSve_d_FCWStatus)
  Runnable_OMAP_10ms_sys/2(OMAPve_y_ADAS_ISLCDriverRemind) -> OMAPve_y_ADAS_ISLCDriverRemind/1
  JABSve_g_DbDecSetpoint/1 -> Runnable_OMAP_10ms_sys/53(JABSve_g_DbDecSetpoint)
  ELKSve_y_SignalTStamp/1 -> Runnable_OMAP_10ms_sys/90(ELKSve_y_SignalTStamp)
  IMAPve_g_L0_C1/1 -> Runnable_OMAP_10ms_sys/106(IMAPve_g_L0_C1)
  ELKSve_y_state_ELK_function/1 -> Runnable_OMAP_10ms_sys/79(ELKSve_y_state_ELK_function)
  ELKSve_y_EPS_ELK_Control/1 -> Runnable_OMAP_10ms_sys/87(ELKSve_y_EPS_ELK_Control)
  Runnable_OMAP_10ms_sys/38(OMAPve_y_ADAS_LCAStatusDisplay) -> OMAPve_y_ADAS_LCAStatusDisplay/1
  FDMMve_d_JaFcnConf/1 -> Runnable_OMAP_10ms_sys/1(FDMMve_d_JaFcnConf)
  AEBSve_d_MDDdecRequest/1 -> Runnable_OMAP_10ms_sys/32(AEBSve_d_MDDdecRequest)
  Runnable_OMAP_10ms_sys/48(OMAPve_y_ADAS_ICAStatusIcon) -> OMAPve_y_ADAS_ICAStatusIcon/1
  Runnable_OMAP_10ms_sys/36(OMAPve_y_ADAS_LKASwitchState) -> OMAPve_y_ADAS_LKASwitchState/1
  Runnable_OMAP_10ms_sys/33(OMAPve_y_ADAS_LDWStatusDisplay) -> OMAPve_y_ADAS_LDWStatusDisplay/1
  AEBSve_g_DecSetpoint/1 -> Runnable_OMAP_10ms_sys/31(AEBSve_g_DecSetpoint)
  Runnable_OMAP_10ms_sys/1(OMAPve_y_ADAS_ISLCState) -> OMAPve_y_ADAS_ISLCState/1
  AEBSve_d_JABS_Tips/1 -> Runnable_OMAP_10ms_sys/50(AEBSve_d_JABS_Tips)
  Runnable_OMAP_10ms_sys/51(OMAPve_y_ADAS_ESAFaultSt) -> OMAPve_y_ADAS_ESAFaultSt/1
  JABSve_d_DbMDDdecType/1 -> Runnable_OMAP_10ms_sys/55(JABSve_d_DbMDDdecType)
  IMAPva_g_obj_pos_x/1 -> Runnable_OMAP_10ms_sys/103(IMAPva_g_obj_pos_x)
  IMAPve_g_L0_C2/1 -> Runnable_OMAP_10ms_sys/107(IMAPve_g_L0_C2)
  ACCSve_d_ACC_ESCHoldReq/1 -> Runnable_OMAP_10ms_sys/24(ACCSve_d_ACC_ESCHoldReq)
  LKASve_g_EPS_Factor_Control/1 -> Runnable_OMAP_10ms_sys/75(LKASve_g_EPS_Factor_Control)
  IMAPve_g_R0_C1/1 -> Runnable_OMAP_10ms_sys/110(IMAPve_g_R0_C1)
  LKASve_y_HMI_Popup_Status/1 -> Runnable_OMAP_10ms_sys/72(LKASve_y_HMI_Popup_Status)
  FDMMve_d_EwFcnConf/1 -> Runnable_OMAP_10ms_sys/8(FDMMve_d_EwFcnConf)
  Runnable_OMAP_10ms_sys/56(OMAPve_y_ADAS_LightControlValid) -> OMAPve_y_ADAS_LightControlValid/1
  AEBSve_d_Prefill_request/1 -> Runnable_OMAP_10ms_sys/29(AEBSve_d_Prefill_request)
  Runnable_OMAP_10ms_sys/22(OMAPve_y_ADAS_ESCDriveOff) -> OMAPve_y_ADAS_ESCDriveOff/1
  Runnable_OMAP_10ms_sys/32(OMAPve_y_ADAS_LDWWarningSt) -> OMAPve_y_ADAS_LDWWarningSt/1
  AEBSve_d_AEBFaultStatus/1 -> Runnable_OMAP_10ms_sys/41(AEBSve_d_AEBFaultStatus)
  FDMMve_d_ElkFcnConf/1 -> Runnable_OMAP_10ms_sys/4(FDMMve_d_ElkFcnConf)
  LKASve_y_LKA_Action_Indication/1 -> Runnable_OMAP_10ms_sys/71(LKASve_y_LKA_Action_Indication)
  ICABve_d_SignalTStamp/1 -> Runnable_OMAP_10ms_sys/93(ICABve_d_SignalTStamp)
  ACCSve_d_CIPV_ID/1 -> Runnable_OMAP_10ms_sys/16(ACCSve_d_CIPV_ID)
  ICABve_d_ICAState/1 -> Runnable_OMAP_10ms_sys/97(ICABve_d_ICAState)
  ACCSve_d_ACC_ICA_Flag/1 -> Runnable_OMAP_10ms_sys/22(ACCSve_d_ACC_ICA_Flag)
  Runnable_OMAP_10ms_sys/53(OMAPve_y_ADAS_HWAActionSts) -> OMAPve_y_ADAS_HWAActionSts/1
  AEBSve_d_JABS_HapticAlarm/1 -> Runnable_OMAP_10ms_sys/49(AEBSve_d_JABS_HapticAlarm)
  Runnable_OMAP_10ms_sys/9(OMAPve_y_ADAS_ACCMessagePrompt) -> OMAPve_y_ADAS_ACCMessagePrompt/1
  FDMMve_d_AccFcnConf/1 -> Runnable_OMAP_10ms_sys/7(FDMMve_d_AccFcnConf)
  ACCSve_d_ACCMessagePrompt/1 -> Runnable_OMAP_10ms_sys/26(ACCSve_d_ACCMessagePrompt)
  IMAPve_g_ESC_LonAcc/1 -> Runnable_OMAP_10ms_sys/101(IMAPve_g_ESC_LonAcc)
  AEBSve_d_ESCDriveOff/1 -> Runnable_OMAP_10ms_sys/34(AEBSve_d_ESCDriveOff)
  IMAPve_g_R0_C3/1 -> Runnable_OMAP_10ms_sys/112(IMAPve_g_R0_C3)
  ICABve_d_LKATorqueReq/1 -> Runnable_OMAP_10ms_sys/98(ICABve_d_LKATorqueReq)
  ACCSve_d_ACC_DecFlag/1 -> Runnable_OMAP_10ms_sys/15(ACCSve_d_ACC_DecFlag)
  ELKSve_g_ELK_SWA_Control/1 -> Runnable_OMAP_10ms_sys/85(ELKSve_g_ELK_SWA_Control)
  ACCSve_g_ACC_DecReq/1 -> Runnable_OMAP_10ms_sys/14(ACCSve_g_ACC_DecReq)
  Runnable_OMAP_10ms_sys/35(OMAPve_y_ADAS_LKAStatusDisplay) -> OMAPve_y_ADAS_LKAStatusDisplay/1
  JABSve_d_DbFunFARCSta/1 -> Runnable_OMAP_10ms_sys/52(JABSve_d_DbFunFARCSta)
  IMAPve_g_R0_C2/1 -> Runnable_OMAP_10ms_sys/111(IMAPve_g_R0_C2)
  Runnable_OMAP_10ms_sys/19(OMAPve_g_ADAS_DecelerationSet) -> OMAPve_g_ADAS_DecelerationSet/1
  ELKSve_y_EPS_State_Control/1 -> Runnable_OMAP_10ms_sys/84(ELKSve_y_EPS_State_Control)
  AEBSve_d_Braking_progress/1 -> Runnable_OMAP_10ms_sys/37(AEBSve_d_Braking_progress)
  JABSve_d_DbBraking_progress/1 -> Runnable_OMAP_10ms_sys/57(JABSve_d_DbBraking_progress)
  AEBSve_d_SignalTStamp/1 -> Runnable_OMAP_10ms_sys/44(AEBSve_d_SignalTStamp)
  ACCSve_d_VelocitySet/1 -> Runnable_OMAP_10ms_sys/19(ACCSve_d_VelocitySet)
  Runnable_OMAP_10ms_sys/15(OMAPve_y_ADAS_TorqueActivReq) -> OMAPve_y_ADAS_TorqueActivReq/1
  AEBSve_d_JABS_AlertSign/1 -> Runnable_OMAP_10ms_sys/45(AEBSve_d_JABS_AlertSign)
  AEBSve_d_AEBStatus/1 -> Runnable_OMAP_10ms_sys/38(AEBSve_d_AEBStatus)
  AEBSve_d_HapticAlarm/1 -> Runnable_OMAP_10ms_sys/36(AEBSve_d_HapticAlarm)
  AEBSve_d_AEBAlertReq/1 -> Runnable_OMAP_10ms_sys/42(AEBSve_d_AEBAlertReq)
  LKASve_g_LKA_SWA_Control/1 -> Runnable_OMAP_10ms_sys/74(LKASve_g_LKA_SWA_Control)
  JABSve_d_DbAlertReq/1 -> Runnable_OMAP_10ms_sys/62(JABSve_d_DbAlertReq)
  ACCSve_d_ACC_EPBReq/1 -> Runnable_OMAP_10ms_sys/25(ACCSve_d_ACC_EPBReq)
  JABSve_d_DbESCDriveOff/1 -> Runnable_OMAP_10ms_sys/64(JABSve_d_DbESCDriveOff)
  AEBSve_d_functionFARCState/1 -> Runnable_OMAP_10ms_sys/30(AEBSve_d_functionFARCState)
  JABSve_d_DbPrefillReq/1 -> Runnable_OMAP_10ms_sys/51(JABSve_d_DbPrefillReq)
  Runnable_OMAP_10ms_sys/3(OMAPve_y_ADAS_ACCHeadwayDisplay) -> OMAPve_y_ADAS_ACCHeadwayDisplay/1
  JABSve_d_DbSwitchStatus/1 -> Runnable_OMAP_10ms_sys/60(JABSve_d_DbSwitchStatus)
  LKASve_y_LDW_Status_Display/1 -> Runnable_OMAP_10ms_sys/67(LKASve_y_LDW_Status_Display)
  LKASve_y_Hands_Off_Warning/1 -> Runnable_OMAP_10ms_sys/70(LKASve_y_Hands_Off_Warning)
  ACCSve_d_ACC_ESCDriveOff/1 -> Runnable_OMAP_10ms_sys/23(ACCSve_d_ACC_ESCDriveOff)
  JABSve_d_DbSignalTStamp/1 -> Runnable_OMAP_10ms_sys/58(JABSve_d_DbSignalTStamp)
  IMAPve_g_L0_C0/1 -> Runnable_OMAP_10ms_sys/105(IMAPve_g_L0_C0)
  IMAPve_d_EPS_LKA_State/1 -> Runnable_OMAP_10ms_sys/100(IMAPve_d_EPS_LKA_State)
  LKASve_y_Vehicle_Lane_Display/1 -> Runnable_OMAP_10ms_sys/66(LKASve_y_Vehicle_Lane_Display)
  ELKSve_y_HMI_Popup_Status/1 -> Runnable_OMAP_10ms_sys/83(ELKSve_y_HMI_Popup_Status)
  ACCSve_d_ACC_TqFlag/1 -> Runnable_OMAP_10ms_sys/13(ACCSve_d_ACC_TqFlag)
  JABSve_d_DbMDDdecRequest/1 -> Runnable_OMAP_10ms_sys/54(JABSve_d_DbMDDdecRequest)
  LKASve_y_LDW_Flag/1 -> Runnable_OMAP_10ms_sys/69(LKASve_y_LDW_Flag)
  JABSve_d_DbESCHoldReq/1 -> Runnable_OMAP_10ms_sys/65(JABSve_d_DbESCHoldReq)
  FDMMve_g_Adas2Fapa/1 -> Runnable_OMAP_10ms_sys/9(FDMMve_g_Adas2Fapa)
  JABSve_d_DbJACWStatus/1 -> Runnable_OMAP_10ms_sys/59(JABSve_d_DbJACWStatus)
  LKASve_y_EPS_LKA_Control/1 -> Runnable_OMAP_10ms_sys/76(LKASve_y_EPS_LKA_Control)
  FDMMve_d_SignalTStamp/1 -> Runnable_OMAP_10ms_sys/10(FDMMve_d_SignalTStamp)
  AEBSve_d_AEBSwitchStatus/1 -> Runnable_OMAP_10ms_sys/40(AEBSve_d_AEBSwitchStatus)
  ACCSve_d_ACCActive_Signal/1 -> Runnable_OMAP_10ms_sys/17(ACCSve_d_ACCActive_Signal)
  ELKSve_y_ELK_ELKSts/1 -> Runnable_OMAP_10ms_sys/89(ELKSve_y_ELK_ELKSts)
  ACCSve_d_HeadWaySet/1 -> Runnable_OMAP_10ms_sys/20(ACCSve_d_HeadWaySet)

== system MIL4L3_SW6_V1_20220211/CarMaker/VehicleControl/PowerControl/AM_PwrSupCurrentMor ==
  In : Inport
  A/M_Switch : Constant  Value=0
  Data Type Conversion : DataTypeConversion
  Manu_Value : Constant  Value=0
  Switch : Switch  Criteria=u2 ~= 0
  Out : Outport
  wires:
  Manu_Value/1 -> Data Type Conversion/1
  Data Type Conversion/1 -> Switch/1
  Switch/1 -> Out/1
  In/1 -> Switch/3
  A/M_Switch/1 -> Switch/2

== system MIL4L3_SW6_V1_20220211/CarMaker/VehicleControl/PowerControl/AM_PwrSupVoltageMor ==
  In : Inport
  A/M_Switch : Constant  Value=0
  Data Type Conversion : DataTypeConversion
  Manu_Value : Constant  Value=0
  Switch : Switch  Criteria=u2 ~= 0
  Out : Outport
  wires:
  A/M_Switch/1 -> Switch/2
  In/1 -> Switch/3
  Switch/1 -> Out/1
  Data Type Conversion/1 -> Switch/1
  Manu_Value/1 -> Data Type Conversion/1

== system MIL4L3_SW6_V1_20220211/CarMaker/VehicleControl/PowerControl/KL15_SW2 ==
  KL30_SW : Inport
  KL30_SW_cause : DataTypeConversion  OutDataTypeStr=fixdt(0,3,1,0)
  KL30_SW_causeSwitch : Constant  Value=SignalSelectSwitch
  KL30_SW_cause|Con : Constant  Value=SignalConstant
  KL30_SW_cause|Switch : Switch  Threshold=0.5  SaturateOnIntegerOverflow=on  InputSameDT=on
  ToBus_KL30_SW_cause : Outport
  wires:
  KL30_SW/1 -> KL30_SW_cause|Switch/1
  KL30_SW_cause/1 -> ToBus_KL30_SW_cause/1
  KL30_SW_cause|Switch/1 -> KL30_SW_cause/1
  KL30_SW_cause|Con/1 -> KL30_SW_cause|Switch/3
  KL30_SW_causeSwitch/1 -> KL30_SW_cause|Switch/2

== system MIL4L3_SW6_V1_20220211/CarMaker/VehicleControl/PowerControl/KL30_SW1 ==
  KL30_SW : Inport
  KL30_SW_cause : DataTypeConversion  OutDataTypeStr=fixdt(0,3,1,0)
  KL30_SW_causeSwitch : Constant  Value=SignalSelectSwitch
  KL30_SW_cause|Con : Constant  Value=SignalConstant
  KL30_SW_cause|Switch : Switch  Threshold=0.5  SaturateOnIntegerOverflow=on  InputSameDT=on
  ToBus_KL30_SW_cause : Outport
  wires:
  KL30_SW_causeSwitch/1 -> KL30_SW_cause|Switch/2
  KL30_SW_cause|Con/1 -> KL30_SW_cause|Switch/3
  KL30_SW_cause|Switch/1 -> KL30_SW_cause/1
  KL30_SW_cause/1 -> ToBus_KL30_SW_cause/1
  KL30_SW/1 -> KL30_SW_cause|Switch/1

== system MIL4L3_SW6_V1_20220211/CarMaker/VehicleControl/SDFADataLog/CIPV_ID1 ==
  Add : Sum
  Bus Selector1 : BusSelector  OutputSignals=TrafficObjectId
  Constant : Constant
  Constant1 : Constant  Value=-1
  Define CM Dict93 : CarMaker4SL/Define CM Dict  Commented=on  xname=User.IO.Out.CIPV_ID  xmono=off  xtype=UInt  xdvaplace=None  xnstates=0  xfirststate=0  xinitial=0
  Product : Product
  Read CM Dict2 : CarMaker4SL/Read CM Dict  xname=Sensor.Object.Camare.relvTgt.ObjId  xsync=off
  Relational Operator : RelationalOperator  Operator=~=  OutDataTypeStr=boolean  RndMeth=Nearest
  Terminator2 : Terminator
  TrafficObject : CarMaker4SL/TrafficObject  xname=INPORT  ximode=Object Id
      settings: SourceProductName=CarMaker4SL
  Write CM Dict81 : CarMaker4SL/Write CM Dict  xname=User.IO.Out.CIPV_ID  xsync=off
  Out1 : Outport
  wires:
  TrafficObject/2 -> Bus Selector1/1
  Constant/1 -> Add/1
  Constant1/1 -> Relational Operator/2
  Add/1 -> Product/1
  Product/1 -> Out1/1, Write CM Dict81/1
  TrafficObject/1 -> Terminator2/1
  Bus Selector1/1 -> Add/2  "<TrafficObjectId>"
  Relational Operator/1 -> Product/2
  Read CM Dict2/1 -> Relational Operator/1, TrafficObject/1

== system MIL4L3_SW6_V1_20220211/CarMaker/VehicleControl/SDFADataLog/Subsystem ==
  Constant4 : Constant  Value=0
  Digital Clock : DigitalClock  SampleTime=0.05
  Gain9 : Gain  Gain=20
  Switch : Switch  Threshold=65535
  Out1 : Outport
  wires:
  Digital Clock/1 -> Gain9/1
  Constant4/1 -> Switch/1
  Switch/1 -> Out1/1
  Gain9/1 -> Switch/2, Switch/3

== system MIL4L3_SW6_V1_20220211/CarMaker/VehicleControl/SDFADataLog/Subsystem1 ==
  BusCreator : BusCreator  Inputs=24
  Ground{,1..19} (20 alike) : Ground
  Read CM Dict : CarMaker4SL/Read CM Dict  xname=User.IO.Out.LongDistance_00  xsync=off
  Read CM Dict1 : CarMaker4SL/Read CM Dict  xname=User.IO.Out.LongDistance_01  xsync=off
  Read CM Dict2 : CarMaker4SL/Read CM Dict  xname=User.IO.Out.LongDistance_02  xsync=off
  Read CM Dict3 : CarMaker4SL/Read CM Dict  xname=User.IO.Out.LongDistance_03  xsync=off
  LongDistance : Outport
  wires:
  BusCreator/1 -> LongDistance/1
  Read CM Dict/1 -> BusCreator/1
  Read CM Dict1/1 -> BusCreator/2
  Read CM Dict2/1 -> BusCreator/3
  Read CM Dict3/1 -> BusCreator/4
  Ground/1 -> BusCreator/5
  Ground1/1 -> BusCreator/6
  Ground2/1 -> BusCreator/7
  Ground3/1 -> BusCreator/8
  Ground4/1 -> BusCreator/9
  Ground5/1 -> BusCreator/10
  Ground6/1 -> BusCreator/11
  Ground7/1 -> BusCreator/12
  Ground8/1 -> BusCreator/13
  Ground9/1 -> BusCreator/14
  Ground10/1 -> BusCreator/15
  Ground11/1 -> BusCreator/16
  Ground14/1 -> BusCreator/17
  Ground15/1 -> BusCreator/18
  Ground16/1 -> BusCreator/19
  Ground17/1 -> BusCreator/20
  Ground12/1 -> BusCreator/21
  Ground13/1 -> BusCreator/22
  Ground18/1 -> BusCreator/23
  Ground19/1 -> BusCreator/24

== system MIL4L3_SW6_V1_20220211/CarMaker/VehicleControl/SDFADataLog/Subsystem10 ==
  Bus Creator : BusCreator  Inputs=20
  Ground{,1..15} (16 alike) : Ground
  Read CM Dict : CarMaker4SL/Read CM Dict  xname=User.IO.Out.IFC_obj01_PhiBottom  xsync=off
  Read CM Dict1 : CarMaker4SL/Read CM Dict  xname=User.IO.Out.IFC_obj02_PhiBottom  xsync=off
  Read CM Dict2 : CarMaker4SL/Read CM Dict  xname=User.IO.Out.IFC_obj03_PhiBottom  xsync=off
  Read CM Dict3 : CarMaker4SL/Read CM Dict  xname=User.IO.Out.IFC_obj04_PhiBottom  xsync=off
  obj_PhiBottom : Outport
  wires:
  Read CM Dict2/1 -> Bus Creator/3
  Ground8/1 -> Bus Creator/13
  Ground5/1 -> Bus Creator/10
  Ground9/1 -> Bus Creator/14
  Ground4/1 -> Bus Creator/9
  Read CM Dict3/1 -> Bus Creator/4
  Ground7/1 -> Bus Creator/12
  Ground/1 -> Bus Creator/5
  Ground2/1 -> Bus Creator/7
  Ground13/1 -> Bus Creator/18
  Ground10/1 -> Bus Creator/15
  Ground6/1 -> Bus Creator/11
  Read CM Dict/1 -> Bus Creator/1
  Read CM Dict1/1 -> Bus Creator/2
  Ground1/1 -> Bus Creator/6
  Ground3/1 -> Bus Creator/8
  Ground12/1 -> Bus Creator/17
  Ground14/1 -> Bus Creator/19
  Ground11/1 -> Bus Creator/16
  Ground15/1 -> Bus Creator/20
  Bus Creator/1 -> obj_PhiBottom/1

== system MIL4L3_SW6_V1_20220211/CarMaker/VehicleControl/SDFADataLog/Subsystem100 ==
  BusCreator : BusCreator  Inputs=10
  Data Type Conversion{1..3,92} (4 alike) : DataTypeConversion  OutDataTypeStr=single
  Ground{,1..5} (6 alike) : Ground
  Read CM Dict1 : CarMaker4SL/Read CM Dict  xname=User.IO.Out.ClassHighestProb_S0_002  xsync=off
  Read CM Dict2 : CarMaker4SL/Read CM Dict  xname=User.IO.Out.ClassHighestProb_S0_003  xsync=off
  Read CM Dict3 : CarMaker4SL/Read CM Dict  xname=User.IO.Out.ClassHighestProb_S0_004  xsync=off
  Read CM Dict5 : CarMaker4SL/Read CM Dict  xname=User.IO.Out.ClassHighestProb_S0_001  xsync=off
  LBtar_ClassHighestProb : Outport
  wires:
  Data Type Conversion92/1 -> BusCreator/1
  Data Type Conversion3/1 -> BusCreator/4
  Data Type Conversion2/1 -> BusCreator/3
  Data Type Conversion1/1 -> BusCreator/2
  BusCreator/1 -> LBtar_ClassHighestProb/1
  Read CM Dict3/1 -> Data Type Conversion3/1
  Read CM Dict2/1 -> Data Type Conversion2/1
  Read CM Dict1/1 -> Data Type Conversion1/1
  Read CM Dict5/1 -> Data Type Conversion92/1
  Ground/1 -> BusCreator/5
  Ground1/1 -> BusCreator/6
  Ground2/1 -> BusCreator/7
  Ground3/1 -> BusCreator/8
  Ground4/1 -> BusCreator/9
  Ground5/1 -> BusCreator/10

== system MIL4L3_SW6_V1_20220211/CarMaker/VehicleControl/SDFADataLog/Subsystem103 ==
  BusCreator : BusCreator  Inputs=10
  Data Type Conversion{1..3,92} (4 alike) : DataTypeConversion  OutDataTypeStr=single
  Ground{,1..5} (6 alike) : Ground
  Read CM Dict1 : CarMaker4SL/Read CM Dict  xname=User.IO.Out.ClassHighestProb_S1_002  xsync=off
  Read CM Dict2 : CarMaker4SL/Read CM Dict  xname=User.IO.Out.ClassHighestProb_S1_003  xsync=off
  Read CM Dict3 : CarMaker4SL/Read CM Dict  xname=User.IO.Out.ClassHighestProb_S1_004  xsync=off
  Read CM Dict5 : CarMaker4SL/Read CM Dict  xname=User.IO.Out.ClassHighestProb_S1_001  xsync=off
  RBtar_ClassHighestProb : Outport
  wires:
  Data Type Conversion2/1 -> BusCreator/3
  Data Type Conversion92/1 -> BusCreator/1
  Data Type Conversion3/1 -> BusCreator/4
  Data Type Conversion1/1 -> BusCreator/2
  Ground5/1 -> BusCreator/10
  Ground4/1 -> BusCreator/9
  Ground3/1 -> BusCreator/8
  Ground2/1 -> BusCreator/7
  Ground1/1 -> BusCreator/6
  Ground/1 -> BusCreator/5
  Read CM Dict5/1 -> Data Type Conversion92/1
  Read CM Dict1/1 -> Data Type Conversion1/1
  Read CM Dict2/1 -> Data Type Conversion2/1
  Read CM Dict3/1 -> Data Type Conversion3/1
  BusCreator/1 -> RBtar_ClassHighestProb/1

== system MIL4L3_SW6_V1_20220211/CarMaker/VehicleControl/SDFADataLog/Subsystem107 ==
  BusCreator : BusCreator  Inputs=10
  Data Type Conversion{1..3,144} (4 alike) : DataTypeConversion  OutDataTypeStr=uint16
  Ground{,1..5} (6 alike) : Ground
  Read CM Dict1 : CarMaker4SL/Read CM Dict  xname=User.IO.Out.Id_S1_002  xsync=off
  Read CM Dict2 : CarMaker4SL/Read CM Dict  xname=User.IO.Out.Id_S1_003  xsync=off
  Read CM Dict3 : CarMaker4SL/Read CM Dict  xname=User.IO.Out.Id_S1_004  xsync=off
  Read CM Dict5 : CarMaker4SL/Read CM Dict  xname=User.IO.Out.Id_S1_001  xsync=off
  RBtar_id : Outport
  wires:
  Data Type Conversion3/1 -> BusCreator/4
  Data Type Conversion2/1 -> BusCreator/3
  Data Type Conversion1/1 -> BusCreator/2
  Data Type Conversion144/1 -> BusCreator/1
  BusCreator/1 -> RBtar_id/1
  Read CM Dict3/1 -> Data Type Conversion3/1
  Read CM Dict2/1 -> Data Type Conversion2/1
  Read CM Dict1/1 -> Data Type Conversion1/1
  Read CM Dict5/1 -> Data Type Conversion144/1
  Ground/1 -> BusCreator/5
  Ground1/1 -> BusCreator/6
  Ground2/1 -> BusCreator/7
  Ground3/1 -> BusCreator/8
  Ground4/1 -> BusCreator/9
  Ground5/1 -> BusCreator/10

== system MIL4L3_SW6_V1_20220211/CarMaker/VehicleControl/SDFADataLog/Subsystem108 ==
  BusCreator : BusCreator  Inputs=10
  Data Type Conversion{1..3,92} (4 alike) : DataTypeConversion  OutDataTypeStr=single
  Ground{,1..5} (6 alike) : Ground
  Read CM Dict1 : CarMaker4SL/Read CM Dict  xname=User.IO.Out.XPos_S1_002  xsync=off
  Read CM Dict2 : CarMaker4SL/Read CM Dict  xname=User.IO.Out.XPos_S1_003  xsync=off
  Read CM Dict3 : CarMaker4SL/Read CM Dict  xname=User.IO.Out.XPos_S1_004  xsync=off
  Read CM Dict5 : CarMaker4SL/Read CM Dict  xname=User.IO.Out.XPos_S1_001  xsync=off
  RBtar_Xpos : Outport
  wires:
  Data Type Conversion2/1 -> BusCreator/3
  Data Type Conversion3/1 -> BusCreator/4
  Data Type Conversion92/1 -> BusCreator/1
  Data Type Conversion1/1 -> BusCreator/2
  Ground5/1 -> BusCreator/10
  Ground4/1 -> BusCreator/9
  Ground3/1 -> BusCreator/8
  Ground2/1 -> BusCreator/7
  Ground1/1 -> BusCreator/6
  Ground/1 -> BusCreator/5
  Read CM Dict5/1 -> Data Type Conversion92/1
  Read CM Dict1/1 -> Data Type Conversion1/1
  Read CM Dict2/1 -> Data Type Conversion2/1
  Read CM Dict3/1 -> Data Type Conversion3/1
  BusCreator/1 -> RBtar_Xpos/1

== system MIL4L3_SW6_V1_20220211/CarMaker/VehicleControl/SDFADataLog/Subsystem109 ==
  BusCreator : BusCreator  Inputs=10
  Data Type Conversion{1..3,92} (4 alike) : DataTypeConversion  OutDataTypeStr=single
  Ground{,1..5} (6 alike) : Ground
  Read CM Dict1 : CarMaker4SL/Read CM Dict  xname=User.IO.Out.YPos_S1_002  xsync=off
  Read CM Dict2 : CarMaker4SL/Read CM Dict  xname=User.IO.Out.YPos_S1_003  xsync=off
  Read CM Dict3 : CarMaker4SL/Read CM Dict  xname=User.IO.Out.YPos_S1_004  xsync=off
  Read CM Dict5 : CarMaker4SL/Read CM Dict  xname=User.IO.Out.YPos_S1_001  xsync=off
  RBtar_Ypos : Outport
  wires:
  Data Type Conversion92/1 -> BusCreator/1
  Data Type Conversion2/1 -> BusCreator/3
  Data Type Conversion3/1 -> BusCreator/4
  Data Type Conversion1/1 -> BusCreator/2
  BusCreator/1 -> RBtar_Ypos/1
  Read CM Dict3/1 -> Data Type Conversion3/1
  Read CM Dict2/1 -> Data Type Conversion2/1
  Read CM Dict1/1 -> Data Type Conversion1/1
  Read CM Dict5/1 -> Data Type Conversion92/1
  Ground/1 -> BusCreator/5
  Ground1/1 -> BusCreator/6
  Ground2/1 -> BusCreator/7
  Ground3/1 -> BusCreator/8
  Ground4/1 -> BusCreator/9
  Ground5/1 -> BusCreator/10

== system MIL4L3_SW6_V1_20220211/CarMaker/VehicleControl/SDFADataLog/Subsystem11 ==
  Bus Creator : BusCreator  Inputs=20
  Ground{,1..15} (16 alike) : Ground
  Read CM Dict : CarMaker4SL/Read CM Dict  xname=User.IO.Out.IFC_obj01_Rel_VyStdDevValid  xsync=off
  Read CM Dict1 : CarMaker4SL/Read CM Dict  xname=User.IO.Out.IFC_obj02_Rel_VyStdDevValid  xsync=off
  Read CM Dict2 : CarMaker4SL/Read CM Dict  xname=User.IO.Out.IFC_obj03_Rel_VyStdDevValid  xsync=off
  Read CM Dict3 : CarMaker4SL/Read CM Dict  xname=User.IO.Out.IFC_obj04_Rel_VyStdDevValid  xsync=off
  obj_Rel_VyStdDevValid : Outport
  wires:
  Read CM Dict2/1 -> Bus Creator/3
  Ground8/1 -> Bus Creator/13
  Ground5/1 -> Bus Creator/10
  Ground9/1 -> Bus Creator/14
  Ground4/1 -> Bus Creator/9
  Read CM Dict3/1 -> Bus Creator/4
  Ground7/1 -> Bus Creator/12
  Ground/1 -> Bus Creator/5
  Ground2/1 -> Bus Creator/7
  Ground13/1 -> Bus Creator/18
  Ground10/1 -> Bus Creator/15
  Ground6/1 -> Bus Creator/11
  Read CM Dict/1 -> Bus Creator/1
  Read CM Dict1/1 -> Bus Creator/2
  Ground1/1 -> Bus Creator/6
  Ground3/1 -> Bus Creator/8
  Ground12/1 -> Bus Creator/17
  Ground14/1 -> Bus Creator/19
  Ground11/1 -> Bus Creator/16
  Ground15/1 -> Bus Creator/20
  Bus Creator/1 -> obj_Rel_VyStdDevValid/1

== system MIL4L3_SW6_V1_20220211/CarMaker/VehicleControl/SDFADataLog/Subsystem110 ==
  BusCreator : BusCreator  Inputs=10
  Data Type Conversion{1..3,92} (4 alike) : DataTypeConversion  OutDataTypeStr=single
  Ground{,1..5} (6 alike) : Ground
  Read CM Dict1 : CarMaker4SL/Read CM Dict  xname=User.IO.Out.XVelocity_S1_002  xsync=off
  Read CM Dict2 : CarMaker4SL/Read CM Dict  xname=User.IO.Out.XVelocity_S1_003  xsync=off
  Read CM Dict3 : CarMaker4SL/Read CM Dict  xname=User.IO.Out.XVelocity_S1_004  xsync=off
  Read CM Dict5 : CarMaker4SL/Read CM Dict  xname=User.IO.Out.XVelocity_S1_001  xsync=off
  RBtar_Xvelocity : Outport
  wires:
  Data Type Conversion92/1 -> BusCreator/1
  Data Type Conversion3/1 -> BusCreator/4
  Data Type Conversion2/1 -> BusCreator/3
  Data Type Conversion1/1 -> BusCreator/2
  Ground5/1 -> BusCreator/10
  Ground4/1 -> BusCreator/9
  Ground3/1 -> BusCreator/8
  Ground2/1 -> BusCreator/7
  Ground1/1 -> BusCreator/6
  Ground/1 -> BusCreator/5
  Read CM Dict5/1 -> Data Type Conversion92/1
  Read CM Dict1/1 -> Data Type Conversion1/1
  Read CM Dict2/1 -> Data Type Conversion2/1
  Read CM Dict3/1 -> Data Type Conversion3/1
  BusCreator/1 -> RBtar_Xvelocity/1

== system MIL4L3_SW6_V1_20220211/CarMaker/VehicleControl/SDFADataLog/Subsystem111 ==
  BusCreator : BusCreator  Inputs=10
  Data Type Conversion{1..3,92} (4 alike) : DataTypeConversion  OutDataTypeStr=single
  Ground{,1..5} (6 alike) : Ground
  Read CM Dict1 : CarMaker4SL/Read CM Dict  xname=User.IO.Out.YVelocity_S1_002  xsync=off
  Read CM Dict2 : CarMaker4SL/Read CM Dict  xname=User.IO.Out.YVelocity_S1_003  xsync=off
  Read CM Dict3 : CarMaker4SL/Read CM Dict  xname=User.IO.Out.YVelocity_S1_004  xsync=off
  Read CM Dict5 : CarMaker4SL/Read CM Dict  xname=User.IO.Out.YVelocity_S1_001  xsync=off
  RBtar_Yvelocity : Outport
  wires:
  Data Type Conversion3/1 -> BusCreator/4
  Data Type Conversion1/1 -> BusCreator/2
  Data Type Conversion2/1 -> BusCreator/3
  Data Type Conversion92/1 -> BusCreator/1
  BusCreator/1 -> RBtar_Yvelocity/1
  Read CM Dict3/1 -> Data Type Conversion3/1
  Read CM Dict2/1 -> Data Type Conversion2/1
  Read CM Dict1/1 -> Data Type Conversion1/1
  Read CM Dict5/1 -> Data Type Conversion92/1
  Ground/1 -> BusCreator/5
  Ground1/1 -> BusCreator/6
  Ground2/1 -> BusCreator/7
  Ground3/1 -> BusCreator/8
  Ground4/1 -> BusCreator/9
  Ground5/1 -> BusCreator/10

== system MIL4L3_SW6_V1_20220211/CarMaker/VehicleControl/SDFADataLog/Subsystem112 ==
  BusCreator : BusCreator  Inputs=10
  Data Type Conversion{1..3,92} (4 alike) : DataTypeConversion  OutDataTypeStr=single
  Ground{,1..5} (6 alike) : Ground
  Read CM Dict1 : CarMaker4SL/Read CM Dict  xname=User.IO.Out.XAcceleration_S1_002  xsync=off
  Read CM Dict2 : CarMaker4SL/Read CM Dict  xname=User.IO.Out.XAcceleration_S1_003  xsync=off
  Read CM Dict3 : CarMaker4SL/Read CM Dict  xname=User.IO.Out.XAcceleration_S1_004  xsync=off
  Read CM Dict5 : CarMaker4SL/Read CM Dict  xname=User.IO.Out.XAcceleration_S1_001  xsync=off
  RBtar_Xacceleration : Outport
  wires:
  Data Type Conversion3/1 -> BusCreator/4
  Data Type Conversion92/1 -> BusCreator/1
  Data Type Conversion2/1 -> BusCreator/3
  Data Type Conversion1/1 -> BusCreator/2
  Ground5/1 -> BusCreator/10
  Ground4/1 -> BusCreator/9
  Ground3/1 -> BusCreator/8
  Ground2/1 -> BusCreator/7
  Ground1/1 -> BusCreator/6
  Ground/1 -> BusCreator/5
  Read CM Dict5/1 -> Data Type Conversion92/1
  Read CM Dict1/1 -> Data Type Conversion1/1
  Read CM Dict2/1 -> Data Type Conversion2/1
  Read CM Dict3/1 -> Data Type Conversion3/1
  BusCreator/1 -> RBtar_Xacceleration/1
